simulink model "model"  (R2020a)
settings: Solver=VariableStepAuto  StartTime=0.0  StopTime=10.0  RelTol=1e-3
values from neighbouring files (symbols this model uses):
  be = 2.0    [data.sldd]    (also in datadict.sldd)
  bv = 1.0    [data.sldd]    (also in datadict.sldd)
  Ie = 1.0    [data.sldd]    (also in datadict.sldd)
  Iv = 5.0    [data.sldd]    (also in datadict.sldd)
settings Model: DataDictionary=data.sldd  OrderedModelArguments=off  Creator=PRATIKSHA  LastModifiedBy=PRATIKSHA

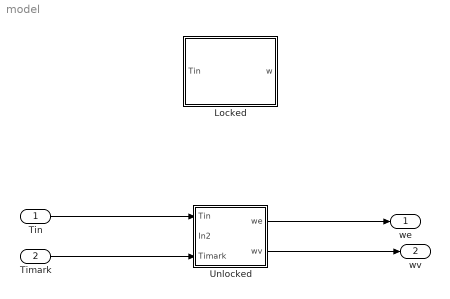
== system model ==
  Tin : Inport
  Timark : Inport  Port=2
  Locked : Subsystem
  Unlocked : Subsystem
  we : Outport
  wv : Outport  Port=2
  wires:
  Tin/1 -> Unlocked/1(Tin)
  Timark/1 -> Unlocked/3(Timark)
  Unlocked/1(we) -> we/1
  Unlocked/2(wv) -> wv/1

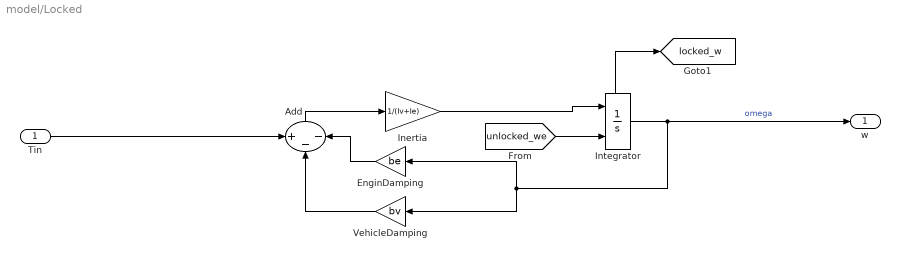
== system model/Locked ==
  Tin : Inport
  " VehicleDamping" : Gain  Gain=bv
  Add : Sum  Inputs=+--
  EnginDamping : Gain  Gain=be
  Inertia : Gain  Gain=1/(Iv+Ie)
  Integrator : Integrator  InitialConditionSource=external  ShowStatePort=on
  w : Outport
  tag scope: locked_w=global
  wires:
  Tin/1 -> Add/1
  Integrator/1 -> w/1, EnginDamping/1, " VehicleDamping"/1  "omega"
  EnginDamping/1 -> Add/3
  Add/1 -> Inertia/1
  [unlocked_we] -> Integrator/2
  " VehicleDamping"/1 -> Add/2
  Inertia/1 -> Integrator/1
  Integrator/State -> [locked_w]

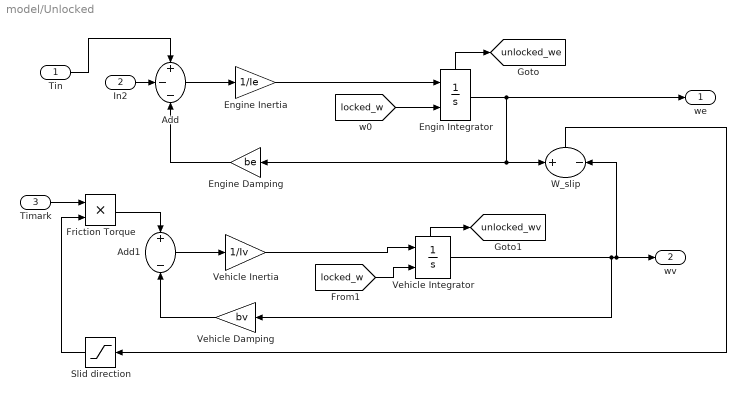
== system model/Unlocked ==
  Tin : Inport
  In2 : Inport  Port=2
  Timark : Inport  Port=3
  Add : Sum  Inputs=+--
  Add1 : Sum  Inputs=+-
  Engin Integrator : Integrator  InitialConditionSource=external  ShowStatePort=on
  Engine Damping : Gain  Gain=be
  Engine Inertia : Gain  Gain=1/Ie
  Friction Torque : Product
  Slid direction : Saturate
  Vehicle Damping : Gain  Gain=bv
  Vehicle Inertia : Gain  Gain=1/Iv
  Vehicle Integrator : Integrator  InitialConditionSource=external  ShowStatePort=on
  W_slip : Sum  Inputs=+-
  we : Outport
  wv : Outport  Port=2
  tag scope: unlocked_we=global, unlocked_wv=global
  wires:
  [locked_w] -> Engin Integrator/2
  Engine Damping/1 -> Add/3
  Friction Torque/1 -> Add1/1
  W_slip/1 -> Slid direction/1
  Vehicle Integrator/1 -> Vehicle Damping/1, wv/1, W_slip/2
  Add/1 -> Engine Inertia/1
  In2/1 -> Add/2
  Engin Integrator/1 -> we/1, W_slip/1, Engine Damping/1
  Add1/1 -> Vehicle Inertia/1
  Engine Inertia/1 -> Engin Integrator/1
  Tin/1 -> Add/1
  Slid direction/1 -> Friction Torque/2
  Vehicle Integrator/State -> [unlocked_wv]
  Vehicle Inertia/1 -> Vehicle Integrator/1
  Timark/1 -> Friction Torque/1
  Vehicle Damping/1 -> Add1/2
  [locked_w] -> Vehicle Integrator/2
  Engin Integrator/State -> [unlocked_we]
